simulink model "BackStepping_Linearization"  (R2019b)
settings: Solver=FixedStepAuto  StartTime=0.0  StopTime=10  FixedStep=0.01  RelTol=1e-3
settings Model: Creator=김태욱  LastModifiedBy=김태욱

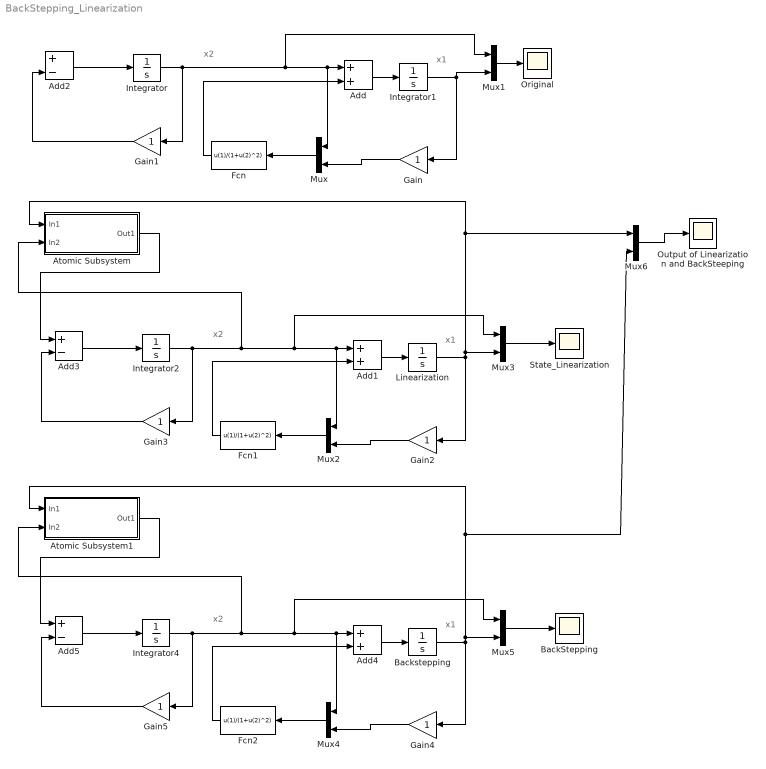
== system BackStepping_Linearization ==
  note: x2
  note: x1
  note: x2
  note: x1
  note: x2
  note: x1
  Add : Sum
  Add1 : Sum
  Add2 : Sum  Inputs=+-
  Add3 : Sum  Inputs=+-
  Add4 : Sum
  Add5 : Sum  Inputs=+-
  Atomic Subsystem : Subsystem  TreatAsAtomicUnit=on
  Atomic Subsystem1 : Subsystem  TreatAsAtomicUnit=on
  BackStepping : Scope
  Backstepping : Integrator  InitialCondition=1
  Fcn : Fcn  Expr=u(1)/(1+u(2)^2)
  Fcn1 : Fcn  Expr=u(1)/(1+u(2)^2)
  Fcn2 : Fcn  Expr=u(1)/(1+u(2)^2)
  Gain{,1..5} (6 alike) : Gain
  Integrator{,1..2,4} (4 alike) : Integrator  InitialCondition=1
  Linearization : Integrator  InitialCondition=1
  Mux{,1..6} (7 alike) : Mux  Inputs=2
  "Original " : Scope
  Output of Linearization and BackSteeping : Scope
  State_Linearization : Scope
  wires:
  Integrator/1 -> Gain1/1, Mux1/1, Mux/1, Add/1
  Add/1 -> Integrator1/1
  Add2/1 -> Integrator/1
  Fcn/1 -> Add/2
  Gain1/1 -> Add2/2
  Gain/1 -> Mux/2
  Mux/1 -> Fcn/1
  Integrator1/1 -> Gain/1, Mux1/2
  Mux1/1 -> "Original "/1
  Mux3/1 -> State_Linearization/1
  Linearization/1 -> Mux6/1, Atomic Subsystem/1(In1), Mux3/2, Gain2/1
  Mux2/1 -> Fcn1/1
  Gain2/1 -> Mux2/2
  Gain3/1 -> Add3/2
  Fcn1/1 -> Add1/2
  Add3/1 -> Integrator2/1
  Add1/1 -> Linearization/1
  Integrator2/1 -> Atomic Subsystem/2(In2), Add1/1, Mux2/1, Mux3/1, Gain3/1
  Atomic Subsystem/1(Out1) -> Add3/1
  Atomic Subsystem1/1(Out1) -> Add5/1
  Integrator4/1 -> Gain5/1, Mux5/1, Mux4/1, Add4/1, Atomic Subsystem1/2(In2)
  Add4/1 -> Backstepping/1
  Add5/1 -> Integrator4/1
  Fcn2/1 -> Add4/2
  Gain5/1 -> Add5/2
  Gain4/1 -> Mux4/2
  Mux4/1 -> Fcn2/1
  Backstepping/1 -> Gain4/1, Mux5/2, Mux6/2, Atomic Subsystem1/1(In1)
  Mux5/1 -> BackStepping/1
  Mux6/1 -> Output of Linearization and BackSteeping/1

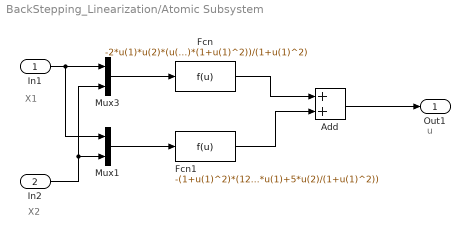
== system BackStepping_Linearization/Atomic Subsystem ==
  note: X1
  note: X2
  note: u
  In1 : Inport
  In2 : Inport  Port=2
  Add : Sum
  Fcn : Fcn  Expr=-2*u(1)*u(2)*(u(1)+u(2)*(1+u(1)^2))/(1+u(1)^2)
  Fcn1 : Fcn  Expr=-(1+u(1)^2)*(12*u(1)+5*u(2)/(1+u(1)^2))
  Mux1 : Mux  Inputs=2
  Mux3 : Mux  Inputs=2
  Out1 : Outport
  wires:
  Add/1 -> Out1/1
  Fcn1/1 -> Add/2
  Fcn/1 -> Add/1
  Mux1/1 -> Fcn1/1
  Mux3/1 -> Fcn/1
  In2/1 -> Mux3/2, Mux1/2
  In1/1 -> Mux3/1, Mux1/1

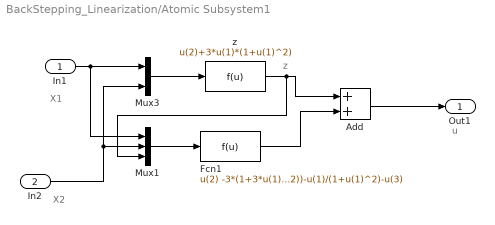
== system BackStepping_Linearization/Atomic Subsystem1 ==
  note: z
  note: u
  note: X2
  note: X1
  In1 : Inport
  In2 : Inport  Port=2
  Add : Sum
  Fcn1 : Fcn  Expr=u(2) -3*(1+3*u(1)^2)*(-2*u(1)+u(3)*(1+u(1)^2))-u(1)/(1+u(1)^2)-u(3)
  Mux1 : Mux  Inputs=3
  Mux3 : Mux  Inputs=2
  z : Fcn  Expr=u(2)+3*u(1)*(1+u(1)^2)
  Out1 : Outport
  wires:
  In1/1 -> Mux1/1, Mux3/1
  In2/1 -> Mux1/2, Mux3/2
  Mux3/1 -> z/1
  Mux1/1 -> Fcn1/1
  z/1 -> Mux1/3, Add/1
  Fcn1/1 -> Add/2
  Add/1 -> Out1/1
